simulink model "chap3_11sim"  (Simulink 5.0)
settings: Solver=ode45  StartTime=0.0  StopTime=20  FixedStep=0.1  RelTol=1e-5
settings Model: LastModifiedBy=Administrator  ExtModeTrigMode=oneshot  ExtModeArmWhenConnect=off  LimitDataPoints=off  BooleanDataType=off

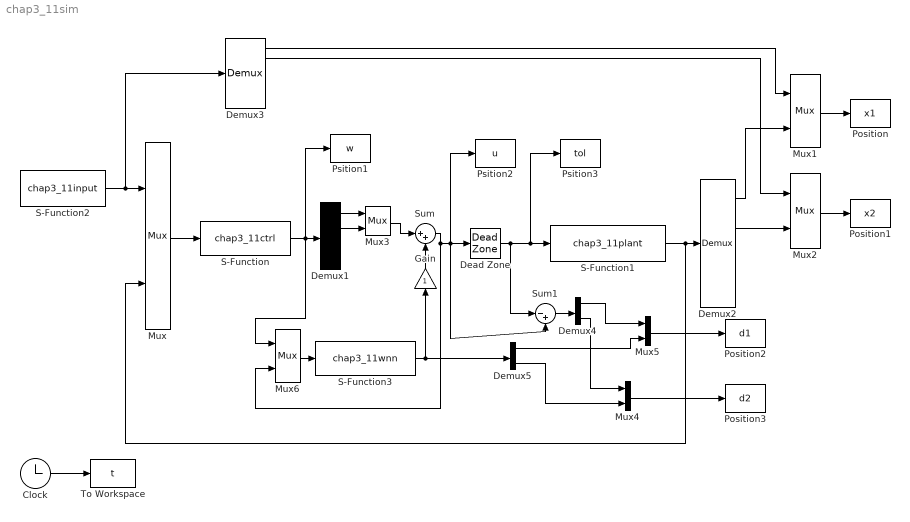
== system chap3_11sim ==
  Clock : Clock
      settings: Decimation=10
  Dead Zone : DeadZone  LowerValue=-10  UpperValue=10  SaturateOnIntegerOverflow=on
  Demux1 : Demux
  Demux2 : Demux
  Demux3 : Demux  Outputs=6
  Demux4 : Demux  Outputs=2
  Demux5 : Demux  Outputs=2
  Gain : Gain  Orientation=up  SaturateOnIntegerOverflow=on
  Mux{,1..6} (7 alike) : Mux  Inputs=2
  Position : ToWorkspace  VariableName=x1  SampleTime=-1  SaveFormat=Array
  Position1 : ToWorkspace  VariableName=x2  SampleTime=-1  SaveFormat=Array
  Position2 : ToWorkspace  VariableName=d1  SampleTime=-1  SaveFormat=Array
  Position3 : ToWorkspace  VariableName=d2  SampleTime=-1  SaveFormat=Array
  Psition1 : ToWorkspace  VariableName=w  SampleTime=-1  SaveFormat=Array
  Psition2 : ToWorkspace  VariableName=u  SampleTime=-1  SaveFormat=Array
  Psition3 : ToWorkspace  VariableName=tol  SampleTime=-1  SaveFormat=Array
  S-Function : S-Function  FunctionName=chap3_11ctrl
  S-Function1 : S-Function  FunctionName=chap3_11plant
  S-Function2 : S-Function  FunctionName=chap3_11input
  S-Function3 : S-Function  FunctionName=chap3_11wnn
  Sum : Sum  Inputs=|++  SaturateOnIntegerOverflow=on
  Sum1 : Sum  Inputs=|-+  SaturateOnIntegerOverflow=on
  To Workspace : ToWorkspace  VariableName=t  SampleTime=-1  SaveFormat=Array
  wires:
  S-Function/1 -> Mux6/1, Demux1/1, Psition1/1
  Demux2/1 -> Mux1/2
  S-Function2/1 -> Demux3/1, Mux/1
  Demux2/2 -> Mux2/2
  Demux3/1 -> Mux1/1
  Demux3/2 -> Mux2/1
  S-Function1/1 -> Mux/2, Demux2/1
  Demux1/1 -> Mux3/1
  Demux1/2 -> Mux3/2
  Dead Zone/1 -> Sum1/1, S-Function1/1, Psition3/1
  Mux3/1 -> Sum/1
  Sum/1 -> Dead Zone/1, Sum1/2, Psition2/1, Mux6/2
  S-Function3/1 -> Gain/1, Demux5/1
  Mux6/1 -> S-Function3/1
  Mux1/1 -> Position/1
  Mux2/1 -> Position1/1
  Mux/1 -> S-Function/1
  Mux5/1 -> Position2/1
  Gain/1 -> Sum/2
  Sum1/1 -> Demux4/1
  Demux4/1 -> Mux5/1
  Demux5/1 -> Mux5/2
  Mux4/1 -> Position3/1
  Demux4/2 -> Mux4/1
  Demux5/2 -> Mux4/2
  Clock/1 -> To Workspace/1
